simulink model "Simulacion_simscape"  (R2018a)
settings: Solver=FixedStepAuto  StartTime=0.0  StopTime=0.001  FixedStep=1e-9  RelTol=1e-3
libraries: fl_lib x13, nesl_utility x6, pe_lib x5, elec_lib x4, pePwmGenerator x4
settings Model: Creator=Tomas  LastModifiedBy=Tomas

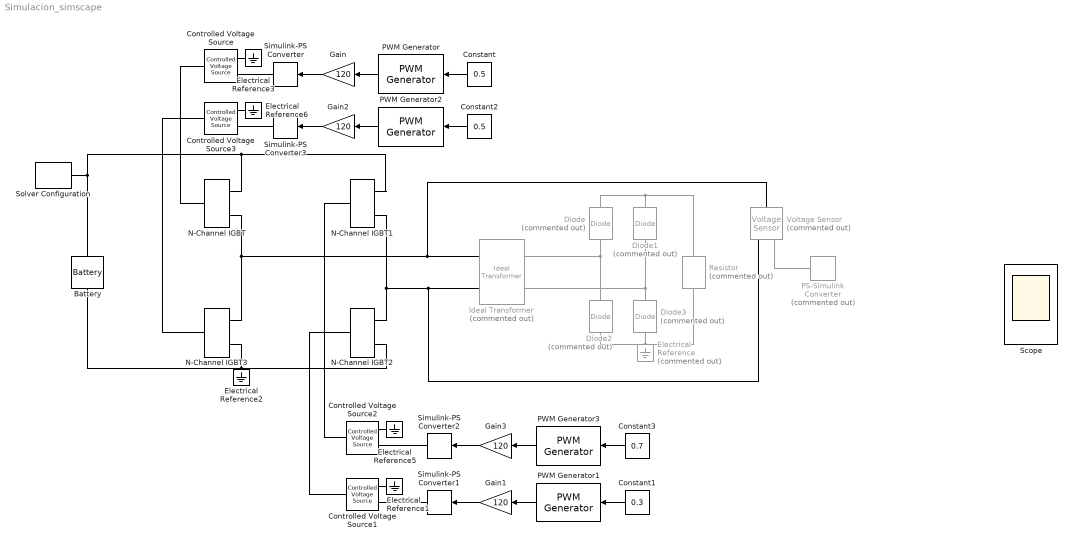
== system Simulacion_simscape ==
  Battery : pe_lib/Sources/Battery  Vnom=110 V  R1=0.54 Ohm  prm_AH=1  AH=50 hr*A  V1=11.5 V  AH1=25 hr*A  prm_R2=1  R2=2000 Ohm  prm_dyn=1  Rp1=0.005 Ohm  tau1=30 s  Rp2=0.005 Ohm  tau2=30 s  prm_fade=1  N_fade=100  AH_fade=45 hr*A  R1_fade=2.02 Ohm  V1_fade=10.35 V  i_specify=off  i_priority=None  i=0 A  i_nominal_specify=off  i_nominal_unit=A  i_nominal_value=1  v_specify=off  v_priority=None  v=0 V  v_nominal_specify=off  v_nominal_unit=V  v_nominal_value=1  charge_specify=off  charge_priority=High  charge=50 hr*A  charge_nominal_specify=off  charge_nominal_unit=hr*A  charge_nominal_value=1  num_cycles_specify=off  num_cycles_priority=High  num_cycles=0  num_cycles_nominal_specify=off  num_cycles_nominal_unit=1  num_cycles_nominal_value=1  thermal_mass=30000 J/K  Tmeas=298.15 K  Vnom_T2=12 V  R1_T2=2.2 Ohm  V1_T2=11.4 V  R2_T2=2200 Ohm  Rp1_T2=0.005 Ohm  tau1_T2=30 s  Rp2_T2=0.005 Ohm  tau2_T2=30 s  Tmeas2=273.15 K  temperature_specify=off  temperature_priority=High  temperature=298.15 K  temperature_nominal_specify=off  temperature_nominal_unit=K  temperature_nominal_value=1
      settings: SourceProductName=Simscape Power Systems  SourceProductBaseCode=PS
  Constant : Constant  Value=0.5
  Constant1 : Constant  Value=0.3
  Constant2 : Constant  Value=0.5
  Constant3 : Constant  Value=0.7
  Controlled Voltage Source{,1..3} (4 alike) : fl_lib/Electrical/Electrical Sources/Controlled Voltage Source
  Diode{,1..3} (4 alike) : pe_lib/Semiconductors/Fundamental Components/Diode  Commented=on  Vf=0.8 V  Ron=0.001 Ohm  Goff=1e-5 1/Ohm  N_series=1  N_parallel=1  Vf_equiv=0.8 V  Ron_equiv=0.001 Ohm  Goff_equiv=1e-5 1/Ohm
      settings: SourceProductName=Simscape Power Systems  SourceProductBaseCode=PS
  Electrical Reference : fl_lib/Electrical/Electrical Elements/Electrical Reference  Commented=on
  Electrical Reference{1..3,5..6} (5 alike) : fl_lib/Electrical/Electrical Elements/Electrical Reference
  Gain{,1..3} (4 alike) : Gain  Gain=120
  Ideal Transformer : fl_lib/Electrical/Electrical Elements/Ideal Transformer  Commented=on  n=1  i1_specify=off  i1_priority=None  i1=0 A  i1_nominal_specify=off  i1_nominal_unit=A  i1_nominal_value=1  v1_specify=off  v1_priority=None  v1=0 V  v1_nominal_specify=off  v1_nominal_unit=V  v1_nominal_value=1  i2_specify=off  i2_priority=None  i2=0 A  i2_nominal_specify=off  i2_nominal_unit=A  i2_nominal_value=1  v2_specify=off  v2_priority=None  v2=0 V  v2_nominal_specify=off  v2_nominal_unit=V  v2_nominal_value=1
      settings: SourceProductName=Simscape  SourceProductBaseCode=SS
  N-Channel IGBT{,1..3} (4 alike) : elec_lib/Semiconductor Devices/N-Channel IGBT  model_type=1  Ices=2 mA  Vces=600 V  Vth=6 V  Vce_sat=2.6 V  Ice_sat=400 A  Vge_sat=10 V  ec=1  Tmeas=25 degC  Vge_vec=[-2, 6, 7, 8, 10, 12, 15, 20] V  Vce_vec=[-1, 0, .5, 1, 1.5, 2, 2.5, 3, 3.5, 4] V  T_vec=[25, 125] degC  Ic_mat=[-1.015e-05, 1.35e-08, .00047135, .0005092, .0005105, .00051175, .00051299, .00051423, .00051548, .00051672; -9.9869e-06, 1.35e-08, .00047135, .0005092, .0005105, .00051175, .00051299, .00051423, .00051548, .00051672; -9.955e-06, 1.35e-08, .0065225, 3.3324, 48.154, 93.661, 105.52, 105.72, 105.93, 106.14; -9.955e-06, 1.35e-08, .0065235, 3.5783, 70.264, 166.33, 252.4, 317.67, 353.38, 357.39; -9.955e-06, 1.35e-08, .006524, 3.7206, 89.171, 228.09, 371.63, 511.02, 642.69, 764.04; -9.9549e-06, 1.35e-08, .0065242, 3.7716, 97.793, 256.21, 424.27, 592.92, 759.2, 921.52; -9.9549e-06, 1.35e-08, .0065243, 3.8067, 104.52, 278.11, 464.6, 654.37, 844.57, 1033.9; -9.9549e-06, 1.35e-08, .0065244, 3.8324, 109.92, 295.67, 496.54, 702.28, 909.96, 1118.3] A  Ic_mat_3D=zeros(8, 10, 2) A  C_param=1  C_GE=23.7 nF  C_GC=2.7 nF  C_CE=0 nF  C_ies=26.4 nF  C_res=2.7 nF  C_oes=0 nF  C_GE_vec=[25, 31, 26.5, 24.9, 25, 24.9, 24.6, 24.7, 24.8] nF  C_GC_vec=[55, 9, 5.5, 3.1, 2.5, 2.1, 1.9, 1.8, 1.7] nF  C_CE_vec=[5, 11, 6.5, 4.9, 3.5, 2.7, 2.1, 1.7, 1.4] nF  C_ies_vec=[80, 40, 32, 28, 27.5, 27, 26.5, 26.5, 26.5] nF  C_res_vec=[55, 9, 5.5, 3.1, 2.5, 2.1, 1.9, 1.8, 1.7] nF  C_oes_vec=[60, 20, 12, 8, 6, 4.8, 4, 3.5, 3.1] nF  C_Vce_vec=[0, 1, 2, 5, 10, 15, 20, 25, 30] V  charge_linearity_param=1  C_OX=20 nF  V_C_OX=-5 V  TF=0 us  VAF=200 V  RC=0.001 Ohm  RE=0.001 Ohm  RG=0.001 Ohm  BF=50  T_param=1  Ices_T2=100 mA  EG=1.11 eV  Vce_sat_T2=3 V  Tmeas2=125 degC  XTI=3  BEX=-1.5  RG_alpha=0 1/K  Tdevice=25 degC  Tdevice_3D=25 degC  Rth=[0, 10] K/W  thermal_mass_parameterization=1  thermal_mass=[0, 1] J/K  thermal_time_constant=[0, 10] s  thermal_mass_initial_temperatures=[298.15, 298.15] K  Ic_vec1=[0, 10, 50, 100, 200, 400, 600] A  Vce_vec1=[0, 1.1, 1.3, 1.45, 1.75, 2.25, 2.7] V  Rmiller=0.1 Ohm  Goff=1e-5 1/Ohm  t_on=0.07 us  t_rise=0.7 us  t_off=0.2 us  t_fall=0.5 us  v_meas=300 V  Tj_vec1=[298.15, 398.15] K  Vce_mat1=[0, 1.1, 1.3, 1.45, 1.75, 2.25, 2.7; 0, 1, 1.15, 1.35, 1.7, 2.35, 3] V  E_turn_on_mat1=[0, .2, 1, 2, 4, 8, 15; 0, .3, 1.3, 2.5, 5, 11, 18] * 1e-3 J  E_turn_off_mat1=[0, .3, 1.5, 3, 6, 15, 25; 0, .7, 3.3, 6.5, 13, 25, 35] * 1e-3 J
      settings: SourceProductName=Simscape Electronics  SourceProductBaseCode=SN
  PS-Simulink Converter : nesl_utility/PS-Simulink Converter  Commented=on  PhysicalDomain=network_engine_domain  SubClassName=ps_output  LeftPortType=input  RightPortType=output  PseudoPeriodic=off  Frequencies=[]  Unit=1  AffineConversion=off
  PWM Generator : pePwmGenerator/PWM Generator  CarrCount=Up  Tper=100e-6  Ts=5e-8
  PWM Generator1 : pePwmGenerator/PWM Generator  CarrCount=Up  Tper=100e-6  Ts=5e-8
  PWM Generator2 : pePwmGenerator/PWM Generator  CarrCount=Down  Tper=100e-6  Ts=5e-8
  PWM Generator3 : pePwmGenerator/PWM Generator  CarrCount=Down  Tper=100e-6  Ts=5e-8
  Resistor : fl_lib/Electrical/Electrical Elements/Resistor  Commented=on  R=1 Ohm  i_specify=off  i_priority=None  i=0 A  i_nominal_specify=off  i_nominal_unit=A  i_nominal_value=1  v_specify=off  v_priority=None  v=0 V  v_nominal_specify=off  v_nominal_unit=V  v_nominal_value=1
  Scope : Scope  NumInputPorts=2
  Simulink-PS Converter{,1..3} (4 alike) : nesl_utility/Simulink-PS Converter  PhysicalDomain=network_engine_domain  SubClassName=ps_input  LeftPortType=input  RightPortType=output  PseudoPeriodic=off  Frequencies=[]  NoiseDistribution=none  NoiseParameters=[]  Unit=V  AffineConversion=off  FilteringAndDerivatives=provide  SimscapeFilterOrder=1  InputFilterTimeConstant=0.001  UdotUserProvided=0
  Solver Configuration : nesl_utility/Solver Configuration  PhysicalDomain=network_engine_domain  SubClassName=solver  LeftPortType=input  RightPortType=generic  Tones=[]  Harmonics=[]  SimulateNoise=off  Profile=off  UseLocalSampling=off  EnableSwitchedLinearOptims=on  FrequencyDomain=off  UseCCode=off  RelTol=0.001  AbsTol=1e-06  MinStep=1e-09  ToWorkspace=off  RevertToSquareIcSolve=off  NumHomotopyIterations=100  PhasorMode=off  PhasorModeNumHarmonics=1  DoDC=off  ResidualTolerance=1e-09  UseLocalSolver=off  LocalSolverChoice=NE_BACKWARD_EULER_ADVANCER  LocalSolverSampleTime=0.001  DoFixedCost=off  MaxNonlinIter=3  MaxModeIter=2  LinearAlgebra=Sparse  EquationFormulation=NE_TIME_EF  DelaysMemoryBudget=1024  AutomaticFiltering=on  FilteringTimeConstant=0.001
  Voltage Sensor : fl_lib/Electrical/Electrical Sensors/Voltage Sensor  Commented=on
  wires:
  Constant/1 -> PWM Generator/1
  PWM Generator/1 -> Gain/1
  PWM Generator1/1 -> Gain1/1
  Constant1/1 -> PWM Generator1/1
  PWM Generator2/1 -> Gain2/1
  Constant2/1 -> PWM Generator2/1
  PWM Generator3/1 -> Gain3/1
  Constant3/1 -> PWM Generator3/1
  Gain3/1 -> Simulink-PS Converter2/1
  Gain1/1 -> Simulink-PS Converter1/1
  Gain/1 -> Simulink-PS Converter/1
  Gain2/1 -> Simulink-PS Converter3/1
  connections:
  N-Channel IGBT/RConn2 -- Voltage Sensor/LConn1 -- Ideal Transformer/LConn1 -- N-Channel IGBT3/RConn1
  N-Channel IGBT3/RConn2 -- Battery/RConn1 -- N-Channel IGBT2/RConn2
  N-Channel IGBT1/RConn2 -- Voltage Sensor/RConn2 -- Ideal Transformer/LConn2 -- N-Channel IGBT2/RConn1
  Diode2/RConn1 -- Ideal Transformer/RConn1 -- Diode/LConn1
  Diode/RConn1 -- Resistor/LConn1 -- Diode1/RConn1
  Diode3/LConn1 -- Electrical Reference/LConn1 -- Diode2/LConn1 -- Resistor/RConn1
  Diode1/LConn1 -- Ideal Transformer/RConn2 -- Diode3/RConn1
  Voltage Sensor/RConn1 -- PS-Simulink Converter/LConn1
  N-Channel IGBT1/RConn1 -- Solver Configuration/RConn1 -- Battery/LConn1 -- N-Channel IGBT/RConn1
  Simulink-PS Converter/RConn1 -- Controlled Voltage Source/RConn1
  Electrical Reference3/LConn1 -- Controlled Voltage Source/RConn2
  Controlled Voltage Source/LConn1 -- N-Channel IGBT/LConn1
  Simulink-PS Converter1/RConn1 -- Controlled Voltage Source1/RConn1
  Electrical Reference1/LConn1 -- Controlled Voltage Source1/RConn2
  Electrical Reference6/LConn1 -- Controlled Voltage Source3/RConn2
  Controlled Voltage Source3/LConn1 -- N-Channel IGBT3/LConn1
  Simulink-PS Converter3/RConn1 -- Controlled Voltage Source3/RConn1
  Controlled Voltage Source2/LConn1 -- N-Channel IGBT1/LConn1
  Simulink-PS Converter2/RConn1 -- Controlled Voltage Source2/RConn1
  Electrical Reference5/LConn1 -- Controlled Voltage Source2/RConn2
  Controlled Voltage Source1/LConn1 -- N-Channel IGBT2/LConn1
